simulink model "F2s1"  (R2020a)
settings: Solver=VariableStepAuto  StartTime=0.0  StopTime=10.0  RelTol=1e-3
settings Model: Creator=User  LastModifiedBy=User

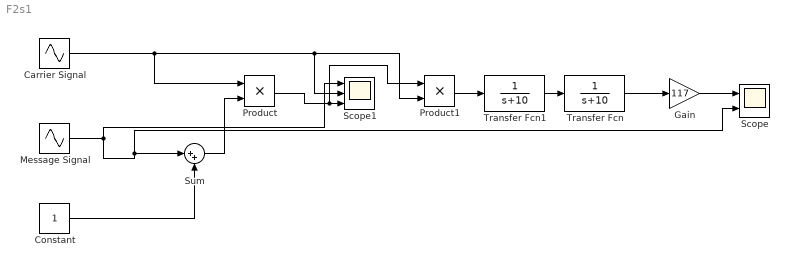
== system F2s1 ==
  Carrier Signal : Sin  Frequency=2*pi*25  SampleTime=1/5000
  Constant : Constant
  Gain : Gain  Gain=117
  Message Signal : Sin  Frequency=2*pi  SampleTime=1/5000
  Product : Product
  Product1 : Product
  Scope : Scope  NumInputPorts=2
  Scope1 : Scope  NumInputPorts=3
  Sum : Sum  Inputs=|++
  Transfer Fcn : TransferFcn  Denominator=[1 10]
  Transfer Fcn1 : TransferFcn  Denominator=[1 10]
  wires:
  Constant/1 -> Sum/2
  Message Signal/1 -> Scope/2, Sum/1, Scope1/1
  Sum/1 -> Product/2
  Carrier Signal/1 -> Product1/2, Scope1/2, Product/1
  Product/1 -> Product1/1, Scope1/3
  Product1/1 -> Transfer Fcn1/1
  Transfer Fcn1/1 -> Transfer Fcn/1
  Transfer Fcn/1 -> Gain/1
  Gain/1 -> Scope/1
